simulink model "model2"  (R2016a)
settings: Solver=VariableStepAuto  StartTime=0.0  StopTime=10.0  MaxStep=1e-3  RelTol=1e-3
undefined symbols (not defined in the file): b, Fe, k, l10, M, m, y0
settings Model: Creator=marek  LastModifiedBy=marek
settings GRTTargetCC: GeneratePreprocessorConditionals=Use local settings

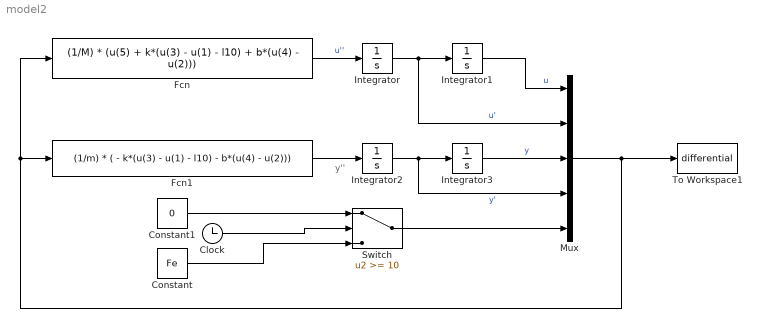
== system model2 ==
  note: y''
  Clock : Clock
  Constant : Constant  Value=Fe
  Constant1 : Constant  Value=0
  Fcn : Fcn  Expr=(1/M) * (u(5) + k*(u(3) - u(1) - l10) + b*(u(4) - u(2)))
  Fcn1 : Fcn  Expr=(1/m) * ( - k*(u(3) - u(1) - l10) - b*(u(4) - u(2)))
  Integrator : Integrator
  Integrator1 : Integrator
  Integrator2 : Integrator
  Integrator3 : Integrator  InitialCondition=y0
  Mux : Mux  Inputs=5
  Switch : Switch  Threshold=10
  To Workspace1 : ToWorkspace  VariableName=differential  SaveFormat=Timeseries  SampleTime=-1
  wires:
  Integrator/1 -> Mux/2, Integrator1/1  "u'"
  Integrator1/1 -> Mux/1  "u"
  Integrator2/1 -> Mux/4, Integrator3/1  "y'"
  Integrator3/1 -> Mux/3  "y"
  Mux/1 -> Fcn1/1, Fcn/1, To Workspace1/1
  Fcn/1 -> Integrator/1  "u''"
  Fcn1/1 -> Integrator2/1
  Switch/1 -> Mux/5
  Clock/1 -> Switch/2
  Constant1/1 -> Switch/1
  Constant/1 -> Switch/3
